simulink model "GoHomeV2"  (R2021b)
settings: Solver=ode23t  StartTime=0.0  StopTime=inf  RelTol=1e-3
InitFcn:
  | RPInit
model workspace (MAT data in the model file):
  mapForSim : object (value not decoded)
  occGrid : robotics.BinaryOccupancyGrid (value not decoded)
undefined symbols (not defined in the file or in its folder): X, Y, Z
libraries: sm_lib x25, nesl_utility x11, RP_Simulator_Components x7, ME598_ProjectLibrary x6, RoboticsPlayground x2, Contact_Forces_Lib x2
(part 2 of 2)

== stateflow chart GoHomeV2/Chart ==
  state DriveToRandLocation
    entry, during:
    LeftM = 127;
    RightM = 50;
  note: Change the Left and Right motor values to anything. As well as the time to go to different places on the arena.
      |
      | Should be fully functional now!
  state DriveForward [commented out]
    LMotor = 100
    RMotor = 100
  state PivotRight [commented out]
    LMotor = -100
    RMotor = 100
  state gohome1
    state PivotLeft1
      entry, during:
      theta = atan2d(0-y,0-x);
      LeftM = -50;
      RightM = 50;
      exit:
      LeftM=0;
      RightM = 0;
    state diff_less
      entry,during:
      inv_diff = diff +360;
      abs1 = abs(diff)
    state DriveForward
      entry:
      after(0.2,sec)
      during:
      LeftM = 80;
      RightM = 80;
      theta = atan2d(0-y,0-x)
    state Reverse
      entry, during:
      LeftM = -60;
      RightM = -60;
      theta = atan2d(0-y,0-x)
      diff = t-theta
    state PivotRight
      entry, during:
      theta = atan2d(0-y,0-x);
      LeftM = 50;
      RightM = -50;
      exit:
      LeftM = 0;
      RightM = 0;
    state diff_great
      entry,during:
      inv_diff = diff -360;
      abs1 = abs(inv_diff)
    state Stop
      LeftM = 0;
      RightM = 0;
    PivotLeft1 -> gohome1.DriveForward : [t>theta-3.5 && t<theta+3.5]
    diff_less -> PivotLeft1 [order 1] : [inv_diff > abs1]
    gohome1.DriveForward -> PivotLeft1 [order 3] : [(t-(theta-3.5)) < 0]
    diff_great -> PivotLeft1 [order 1] : [diff > abs1]
    Reverse -> diff_less [order 2] : [diff < 0]
    diff_less -> gohome1.PivotRight [order 2] : [inv_diff < abs1]
    (default) -> Reverse
    gohome1.DriveForward -> Stop [order 1] : [x > -0.2 && x < 0.2 && y > -0.2 && y < 0.2]
    gohome1.PivotRight -> gohome1.DriveForward : [t > theta -3.5 && t< theta +3.5]
    gohome1.DriveForward -> gohome1.PivotRight [order 2] : [(t-(theta+3.5)) > 0]
    Reverse -> diff_great [order 1] : [diff > 0]
    diff_great -> gohome1.PivotRight [order 2] : [diff < abs1]
  state NotCenter [commented out]
    LMotor = 100;
    RMotor = 100;
  state Centered [commented out]
    LMotor = 0;
    RMotor = 0;
  (default) -> DriveToRandLocation
  (default) -> PivotRight [commented out]
  DriveToRandLocation -> gohome1 : after (9,sec)
  PivotRight -> DriveForward [commented out] : [Red_Distance >0]
  DriveForward -> PivotRight [commented out] : [Red_Distance < 0]
  (default) -> NotCenter [commented out]
  NotCenter -> Centered [commented out] : [XPos>-0.05 && XPos <0.05]
  Centered -> NotCenter [commented out] : [XPos<-0.05 && XPos >0.05]
  data: LeftM output; theta output; RightM output; x input; y input; t input; diff local; inv_diff local; abs1 local

== matlab function GoHomeV2/-180* : 180* ==
  data: deg input; deg output
function deg = degWrap(deg)

% % Convert radians to degrees
% deg = 180/pi * rad;


% Wrap degree value to the range -180* : +180*
for idx = 1:length(deg)
    while deg(idx) < -180
        deg(idx) = deg(idx)+360;
    end
    
    while deg(idx) > 180
        deg(idx) = deg(idx)-360;
    end
end

return

== matlab function GoHomeV2/-180* : 180*1 ==
  data: deg input; deg output
function deg = degWrap(deg)

% % Convert radians to degrees
% deg = 180/pi * rad;


% Wrap degree value to the range -180* : +180*
for idx = 1:length(deg)
    while deg(idx) < -180
        deg(idx) = deg(idx)+360;
    end
    
    while deg(idx) > 180
        deg(idx) = deg(idx)-360;
    end
end

return
